simulink model "multiAgentTest"  (R2021a)
settings: Solver=VariableStepAuto  StartTime=0.0  StopTime=1000  RelTol=1e-3
libraries: rllib x2
settings Model: Creator=Mitch  LastModifiedBy=Mitch

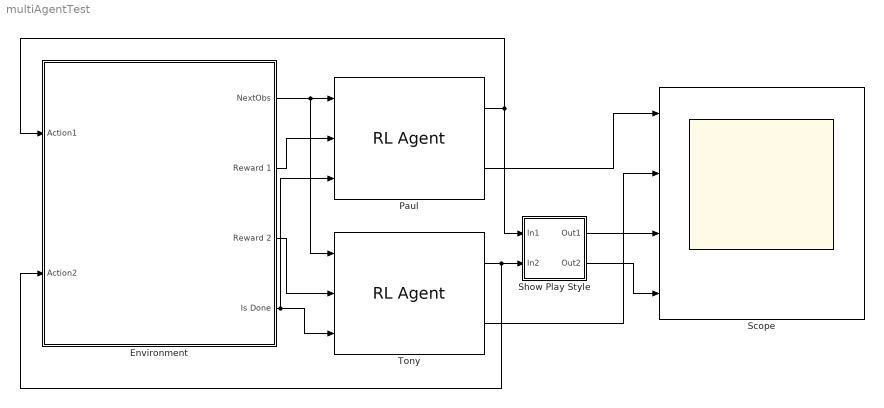
== system multiAgentTest ==
  Environment : Subsystem
  Paul : rllib/RL Agent  Agent=agentPPO  ExternalActionAsInput=off  ProvideCumRwd=on  TreatAsDirectFeedthrough=on
  Scope : Scope  NumInputPorts=4
  Show Play Style : Subsystem
  Tony : rllib/RL Agent  Agent=agentPPO  ExternalActionAsInput=off  ProvideCumRwd=on  TreatAsDirectFeedthrough=on
  wires:
  Tony/2 -> Scope/2
  Paul/2 -> Scope/1
  Environment/1(NextObs) -> Paul/1, Tony/1
  Show Play Style/1(Out1) -> Scope/3
  Show Play Style/2(Out2) -> Scope/4
  Environment/2(Reward 1) -> Paul/2
  Paul/1 -> Environment/1(Action1), Show Play Style/1(In1)
  Environment/3(Reward 2) -> Tony/2
  Tony/1 -> Environment/2(Action2), Show Play Style/2(In2)
  Environment/4(Is Done) -> Paul/3, Tony/3

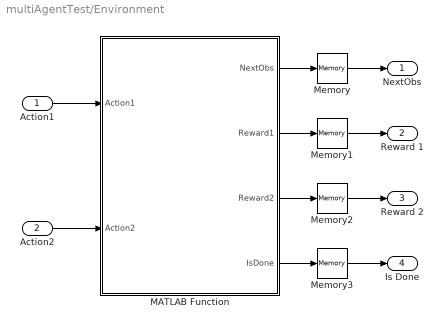
== system multiAgentTest/Environment ==
  Action1 : Inport
  Action2 : Inport  Port=2
  MATLAB Function : MATLAB Function  InitFcn=LoggedSignals = [1; 1];  TreatAsAtomicUnit=on
  Memory : Memory  InitialCondition=[1,1]
  Memory1 : Memory
  Memory2 : Memory
  Memory3 : Memory
  NextObs : Outport
  Reward 1 : Outport  Port=2
  Reward 2 : Outport  Port=3
  Is Done : Outport  Port=4
  wires:
  MATLAB Function/4(IsDone) -> Memory3/1
  MATLAB Function/2(Reward1) -> Memory1/1
  Action2/1 -> MATLAB Function/2(Action2)
  Memory1/1 -> Reward 1/1
  Memory2/1 -> Reward 2/1
  Memory3/1 -> Is Done/1
  Action1/1 -> MATLAB Function/1(Action1)
  MATLAB Function/3(Reward2) -> Memory2/1
  MATLAB Function/1(NextObs) -> Memory/1
  Memory/1 -> NextObs/1

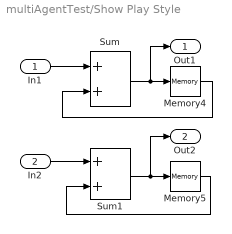
== system multiAgentTest/Show Play Style ==
  In1 : Inport
  In2 : Inport  Port=2
  Memory4 : Memory
  Memory5 : Memory
  Sum : Sum
  Sum1 : Sum
  Out1 : Outport
  Out2 : Outport  Port=2
  wires:
  Memory5/1 -> Sum1/2
  Sum/1 -> Memory4/1, Out1/1
  In1/1 -> Sum/1
  Sum1/1 -> Out2/1, Memory5/1
  Memory4/1 -> Sum/2
  In2/1 -> Sum1/1

== matlab function multiAgentTest/Environment/MATLAB Function ==
  data: Action1 input; NextObs output; Action2 input; Reward1 output; Reward2 output; IsDone output
function [NextObs, Reward1, Reward2, IsDone] = myStepFunction(Action1, Action2)

% Purple 
% Green
%
% C = 1
% D = 2
%
% P P = 1 % Purple on Purple Island
% G G = 1 % Green on Green Island
%
% G P = 3 % Green on Purple Island
% P G = 3 % Purple on Green Island
%
% PG P = 3 + 1 = 4 % Purple and Green on Purple Island
% GP G = 3 + 1 = 4 % Green and Purple on Green Island


% Reward Matrix
%   |  C |  D |
% C | PP | PG |
% D | GP | GG |
%

rewardMatrix = [3, 0; 4, 1];

Reward1 = rewardMatrix(Action1, Action2);
Reward2 = rewardMatrix(Action2, Action1);

NextObs = [Action1, Action2];

IsDone = 0;


end
